simulink model "simlag2"  (Simulink 7.9)
settings: Solver=ode45  StartTime=0.0  StopTime=10.0  RelTol=1e-3
undefined symbols (not defined in the file or in its folder): Ax, Ay, Az, b, g, Ixx, Iyy, Izz, k, l, m
settings Model: Creator=gabriel  LastModifiedBy=gabriel
settings DebuggingCC: SolverPrmCheckMsg=none

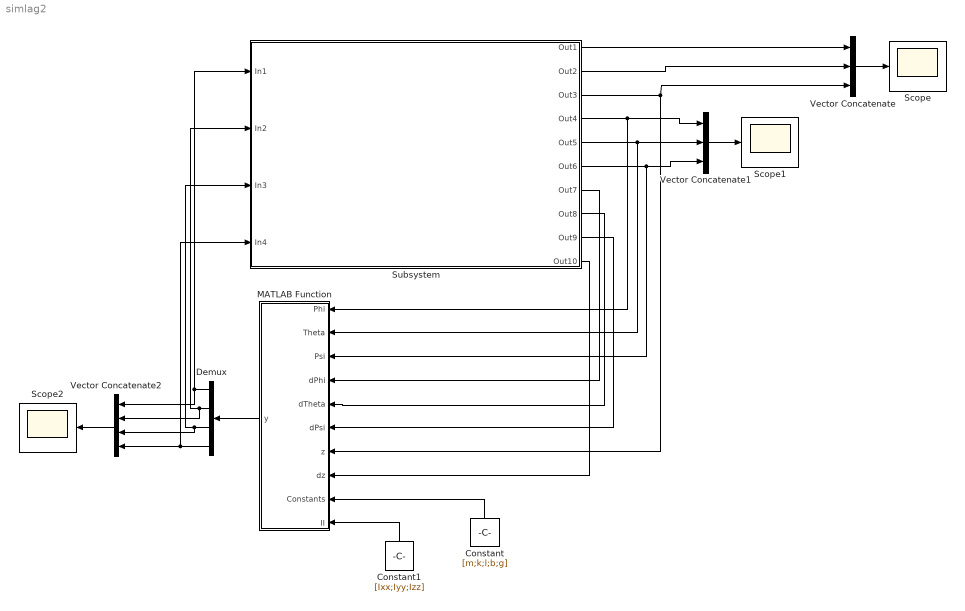
== system simlag2 ==
  Constant : Constant  Value=[m;k;l;b;g]
  Constant1 : Constant  Value=[Ixx;Iyy;Izz]
  Demux : Demux
  MATLAB Function : MATLAB Function  TreatAsAtomicUnit=on
  Scope : Scope
      settings: TickLabels=on  ShowLegends=on
  Scope1 : Scope
      settings: ShowLegends=on
  Scope2 : Scope
      settings: TickLabels=on  ShowLegends=on  SaveName=ScopeData2
  Subsystem : Subsystem
      mask Display: image(imread('Quad.jpeg'))
  Vector Concatenate : Concatenate  NumInputs=3
  Vector Concatenate1 : Concatenate  NumInputs=3
  Vector Concatenate2 : Concatenate  NumInputs=4
  wires:
  Subsystem/1(Out1) -> Vector Concatenate/1
  Subsystem/2(Out2) -> Vector Concatenate/2
  Subsystem/3(Out3) -> Vector Concatenate/3, MATLAB Function/7(z)
  Vector Concatenate/1 -> Scope/1
  Subsystem/4(Out4) -> Vector Concatenate1/1, MATLAB Function/1(Phi)
  Subsystem/5(Out5) -> Vector Concatenate1/2, MATLAB Function/2(Theta)
  Subsystem/6(Out6) -> Vector Concatenate1/3, MATLAB Function/3(Psi)
  Vector Concatenate1/1 -> Scope1/1
  Subsystem/7(Out7) -> MATLAB Function/4(dPhi)
  Subsystem/8(Out8) -> MATLAB Function/5(dTheta)
  Subsystem/9(Out9) -> MATLAB Function/6(dPsi)
  Subsystem/10(Out10) -> MATLAB Function/8(dz)
  Constant/1 -> MATLAB Function/9(Constants)
  Constant1/1 -> MATLAB Function/10(II)
  MATLAB Function/1(y) -> Demux/1
  Demux/1 -> Subsystem/1(In1), Vector Concatenate2/1
  Demux/2 -> Subsystem/2(In2), Vector Concatenate2/2
  Demux/3 -> Subsystem/3(In3), Vector Concatenate2/3
  Demux/4 -> Subsystem/4(In4), Vector Concatenate2/4
  Vector Concatenate2/1 -> Scope2/1

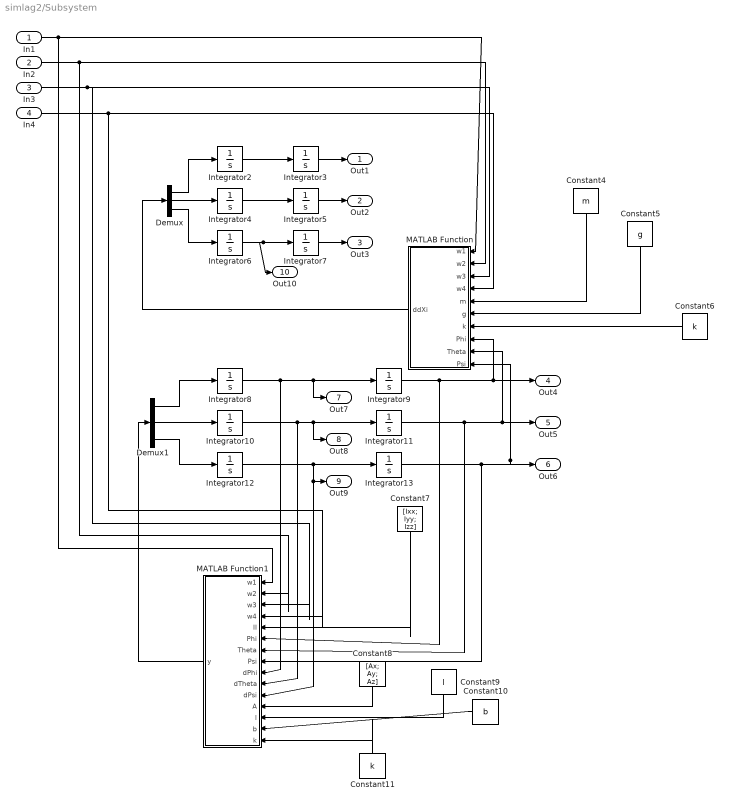
== system simlag2/Subsystem ==
  In1 : Inport
  In2 : Inport  Port=2
  In3 : Inport  Port=3
  In4 : Inport  Port=4
  Constant10 : Constant  Value=b
  Constant11 : Constant  Value=k
  Constant4 : Constant  Value=m
  Constant5 : Constant  Value=g
  Constant6 : Constant  Value=k
  Constant7 : Constant  Value=[Ixx; Iyy; Izz]
  Constant8 : Constant  Value=[Ax; Ay; Az]
  Constant9 : Constant  Value=l
  Demux : Demux  Outputs=3
  Demux1 : Demux  Outputs=3
  Integrator{2..13} (12 alike) : Integrator
  MATLAB Function : MATLAB Function  TreatAsAtomicUnit=on
  MATLAB Function1 : MATLAB Function  TreatAsAtomicUnit=on
  Out1 : Outport
  Out2 : Outport  Port=2
  Out3 : Outport  Port=3
  Out4 : Outport  Port=4
  Out5 : Outport  Port=5
  Out6 : Outport  Port=6
  Out7 : Outport  Port=7
  Out8 : Outport  Port=8
  Out9 : Outport  Port=9
  Out10 : Outport  Port=10
  wires:
  Integrator2/1 -> Integrator3/1
  Integrator4/1 -> Integrator5/1
  Integrator6/1 -> Integrator7/1, Out10/1
  Integrator8/1 -> MATLAB Function1/9(dPhi), Integrator9/1, Out7/1
  Integrator10/1 -> MATLAB Function1/10(dTheta), Integrator11/1, Out8/1
  Integrator12/1 -> Integrator13/1, MATLAB Function1/11(dPsi), Out9/1
  In1/1 -> MATLAB Function/1(w1), MATLAB Function1/1(w1)
  Integrator9/1 -> MATLAB Function1/6(Phi), MATLAB Function/8(Phi), Out4/1
  Integrator11/1 -> MATLAB Function1/7(Theta), MATLAB Function/9(Theta), Out5/1
  Integrator13/1 -> MATLAB Function1/8(Psi), MATLAB Function/10(Psi), Out6/1
  Constant4/1 -> MATLAB Function/5(m)
  Constant5/1 -> MATLAB Function/6(g)
  Constant6/1 -> MATLAB Function/7(k)
  MATLAB Function/1(ddXi) -> Demux/1
  Demux/1 -> Integrator2/1
  Demux/2 -> Integrator4/1
  Demux/3 -> Integrator6/1
  Constant7/1 -> MATLAB Function1/5(II)
  Demux1/1 -> Integrator8/1
  Demux1/2 -> Integrator10/1
  Demux1/3 -> Integrator12/1
  MATLAB Function1/1(y) -> Demux1/1
  Constant8/1 -> MATLAB Function1/12(A)
  Constant9/1 -> MATLAB Function1/13(l)
  Constant10/1 -> MATLAB Function1/14(b)
  Constant11/1 -> MATLAB Function1/15(k)
  Integrator3/1 -> Out1/1
  Integrator5/1 -> Out2/1
  Integrator7/1 -> Out3/1
  In2/1 -> MATLAB Function/2(w2), MATLAB Function1/2(w2)
  In3/1 -> MATLAB Function/3(w3), MATLAB Function1/3(w3)
  In4/1 -> MATLAB Function/4(w4), MATLAB Function1/4(w4)

== matlab function Subsystem/MATLAB Function1 ==
  data: w1 input double; w2 input double; w3 input double; w4 input double; y output double; II input double; Phi input double; Theta input double; Psi input double; dPhi input double; dTheta input double; dPsi input double; A input double; l input double; b input double; k input double
function y = fcn(w1,w2,w3,w4,II,Phi,Theta,Psi,dPhi,dTheta,dPsi,A,l,b,k)
%#codegen

Ixx=II(1);
Iyy=II(2);
Izz=II(3);

% TauB=[[l*k*(w(4)^2-w(2)^2)];
%       [l*k*(w(3)^2-w(1)^2)];
%       [b*(w(1)^2+w(3)^2-w(2)^2-w(4)^2)]];

TauB=[[l*k*(w4-w2)];
      [l*k*(w3-w1)];
      [b*(w1+w3-w2-w4)]];

Weta=[[1 0 -sin(Theta)];
      [0 cos(Phi) cos(Theta)*sin(Phi)];
      [0 -sin(Phi) cos(Theta)*cos(Phi)]];
 
J=transpose(Weta)*[[Ixx 0 0];[0 Iyy 0];[0 0 Izz]]*Weta;  

% CdEta=[((Izz*sin(2*Phi)*cos(Theta)^2)/2 - (Iyy*sin(2*Phi)*cos(Theta)^2)/2)*dPsi^2 + (Izz*cos(2*Phi)*cos(Theta) - Iyy*cos(2*Phi)*cos(Theta) - Ixx*cos(Theta))*dPsi*dTheta + ((Iyy*sin(2*Phi))/2 - (Izz*sin(2*Phi))/2)*dTheta^2;
%        dPsi^2*(Izz*cos(Phi)^2*cos(Theta)*sin(Theta) - Ixx*cos(Theta)*sin(Theta) + Iyy*cos(Theta)*sin(Phi)^2*sin(Theta)) - ddTheta*(Iyy*cos(Phi)^2 + Izz*sin(Phi)^2) - ddPsi*(Iyy*cos(Phi)*cos(Theta)*sin(Phi) - Izz*cos(Phi)*cos(Theta)*sin(Phi)) + Iyy*ddTheta*cos(Phi)^2 + Izz*ddTheta*sin(Phi)^2 - dPhi*dTheta*(2*Iyy*cos(Phi)*sin(Phi) - 2*Izz*cos(Phi)*sin(Phi)) + dPhi*dPsi*(Ixx*cos(Theta) + Iyy*cos(Phi)^2*cos(Theta) - Izz*cos(Phi)^2*cos(Theta) - Iyy*cos(Theta)*sin(Phi)^2 + Izz*cos(Theta)*sin(Phi)^2) + Iyy*ddPsi*cos(Phi)*cos(Theta)*sin(Phi) - Izz*ddPsi*cos(Phi)*cos(Theta)*sin(Phi);
%        Ixx*ddPsi*sin(Theta)^2 - ddPsi*(Izz*cos(Phi)^2*cos(Theta)^2 + Iyy*cos(Theta)^2*sin(Phi)^2 + Ixx*sin(Theta)^2) - ddTheta*(Iyy*cos(Phi)*cos(Theta)*sin(Phi) - Izz*cos(Phi)*cos(Theta)*sin(Phi)) - dTheta^2*(Iyy*cos(Phi)*sin(Phi)*sin(Theta) - Izz*cos(Phi)*sin(Phi)*sin(Theta)) - dPsi*dTheta*(2*Izz*cos(Phi)^2*cos(Theta)*sin(Theta) - 2*Ixx*cos(Theta)*sin(Theta) + 2*Iyy*cos(Theta)*sin(Phi)^2*sin(Theta)) - dPhi*dTheta*(Ixx*cos(Theta) - Iyy*cos(Phi)^2*cos(Theta) + Izz*cos(Phi)^2*cos(Theta) + Iyy*cos(Theta)*sin(Phi)^2 - Izz*cos(Theta)*sin(Phi)^2) + dPhi*dPsi*(2*Iyy*cos(Phi)*cos(Theta)^2*sin(Phi) - 2*Izz*cos(Phi)*cos(Theta)^2*sin(Phi)) + Izz*ddPsi*cos(Phi)^2*cos(Theta)^2 + Iyy*ddPsi*cos(Theta)^2*sin(Phi)^2 + Iyy*ddTheta*cos(Phi)*cos(Theta)*sin(Phi) - Izz*ddTheta*cos(Phi)*cos(Theta)*sin(Phi)]
 
% CdEta=[(Iyy*dTheta^2*sin(2*Phi))/2 - (Izz*dTheta^2*sin(2*Phi))/2 - Ixx*dPsi*dTheta*cos(Theta) - (Iyy*dPsi^2*sin(2*Phi)*cos(Theta)^2)/2 + (Izz*dPsi^2*sin(2*Phi)*cos(Theta)^2)/2 - Iyy*dPsi*dTheta*cos(2*Phi)*cos(Theta) + Izz*dPsi*dTheta*cos(2*Phi)*cos(Theta);
%         dPhi*(Ixx*dPsi*cos(Theta) - 2*Iyy*dTheta*cos(Phi)*sin(Phi) + 2*Izz*dTheta*cos(Phi)*sin(Phi) + Iyy*dPsi*cos(Phi)^2*cos(Theta) - Izz*dPsi*cos(Phi)^2*cos(Theta) - Iyy*dPsi*cos(Theta)*sin(Phi)^2 + Izz*dPsi*cos(Theta)*sin(Phi)^2) - Ixx*dPsi^2*cos(Theta)*sin(Theta) + Iyy*dPsi^2*cos(Theta)*sin(Phi)^2*sin(Theta) + Izz*dPsi^2*cos(Phi)^2*cos(Theta)*sin(Theta);
%         -dPhi*(Ixx*dTheta*cos(Theta) - Iyy*dTheta*cos(Phi)^2*cos(Theta) + Izz*dTheta*cos(Phi)^2*cos(Theta) + Iyy*dTheta*cos(Theta)*sin(Phi)^2 - Izz*dTheta*cos(Theta)*sin(Phi)^2 - 2*Iyy*dPsi*cos(Phi)*cos(Theta)^2*sin(Phi) + 2*Izz*dPsi*cos(Phi)*cos(Theta)^2*sin(Phi))  - Iyy*dTheta^2*cos(Phi)*sin(Phi)*sin(Theta) + Izz*dTheta^2*cos(Phi)*sin(Phi)*sin(Theta) + 2*Ixx*dPsi*dTheta*cos(Theta)*sin(Theta) - 2*Izz*dPsi*dTheta*cos(Phi)^2*cos(Theta)*sin(Theta) - 2*Iyy*dPsi*dTheta*cos(Theta)*sin(Phi)^2*sin(Theta)];    


  CdEta=[(Iyy*dTheta^2*sin(2*Phi))/2 - (Izz*dTheta^2*sin(2*Phi))/2 - Ixx*dPsi*dTheta*cos(Theta) - (Iyy*dPsi^2*sin(2*Phi)*cos(Theta)^2)/2 + (Izz*dPsi^2*sin(2*Phi)*cos(Theta)^2)/2 - Iyy*dPsi*dTheta*cos(2*Phi)*cos(Theta) + Izz*dPsi*dTheta*cos(2*Phi)*cos(Theta);
          dPhi*(Ixx*dPsi*cos(Theta) - 2*Iyy*dTheta*cos(Phi)*sin(Phi) + 2*Izz*dTheta*cos(Phi)*sin(Phi) + Iyy*dPsi*cos(Phi)^2*cos(Theta) - Izz*dPsi*cos(Phi)^2*cos(Theta) - Iyy*dPsi*cos(Theta)*sin(Phi)^2 + Izz*dPsi*cos(Theta)*sin(Phi)^2)  - Ixx*dPsi^2*cos(Theta)*sin(Theta) + Iyy*dPsi^2*cos(Theta)*sin(Phi)^2*sin(Theta)  + Izz*dPsi^2*cos(Phi)^2*cos(Theta)*sin(Theta);
          -dPhi*(Ixx*dTheta*cos(Theta) - Iyy*dTheta*cos(Phi)^2*cos(Theta) + Izz*dTheta*cos(Phi)^2*cos(Theta) + Iyy*dTheta*cos(Theta)*sin(Phi)^2 - Izz*dTheta*cos(Theta)*sin(Phi)^2 - 2*Iyy*dPsi*cos(Phi)*cos(Theta)^2*sin(Phi) + 2*Izz*dPsi*cos(Phi)*cos(Theta)^2*sin(Phi))  - Iyy*dTheta^2*cos(Phi)*sin(Phi)*sin(Theta) + Izz*dTheta^2*cos(Phi)*sin(Phi)*sin(Theta) + 2*Ixx*dPsi*dTheta*cos(Theta)*sin(Theta) - 2*Izz*dPsi*dTheta*cos(Phi)^2*cos(Theta)*sin(Theta) - 2*Iyy*dPsi*dTheta*cos(Theta)*sin(Phi)^2*sin(Theta)];
y = inv(J)*(TauB-CdEta);

== matlab function Subsystem/MATLAB Function ==
  data: w1 input double; w2 input double; w3 input double; w4 input double; m input double; g input double; k input double; Phi input double; Theta input double; Psi input double; ddXi output double
function ddXi = fcn(w1,w2,w3,w4,m,g,k,Phi,Theta,Psi)
%#codegen

R=[[cos(Psi)*cos(Theta) cos(Psi)*sin(Theta)*sin(Phi)-sin(Psi)*cos(Phi) cos(Psi)*sin(Theta)*cos(Phi)+sin(Psi)*sin(Phi)];
   [sin(Psi)*cos(Theta) sin(Psi)*sin(Theta)*sin(Phi)+cos(Psi)*cos(Phi) sin(Psi)*sin(Theta)*cos(Phi)-cos(Psi)*sin(Phi)];
   [-sin(Theta) cos(Theta)*sin(Phi) cos(Theta)*cos(Phi)]];

% T=[0; 0; k*(w(1)^2+w(2)^2+w(3)^2+w(4)^2)/m];

T=[0; 0; k*(w1+w2+w3+w4)/m];

ddXi = R*T+[0; 0; -g];

== matlab function MATLAB Function ==
  data: Phi input double; y output double; Theta input double; Psi input double; dPhi input double; dTheta input double; dPsi input double; z input double; dz input double; Constants input double; II input double
function y = fcn(Phi,Theta,Psi,dPhi,dTheta,dPsi,z,dz,Constants,II)
%#codegen

m=Constants(1);
k=Constants(2);
l=Constants(3);
b=Constants(4);
g=Constants(5);

Ixx=II(1);
Iyy=II(2);
Izz=II(3);

zD=10;
dzD=0;

PhiD=0.5;
ThetaD=0;
PsiD=0;

dPhiD=0;
dThetaD=0;
dPsiD=0;

KphiP=1.5;
KthetaP=6;
KpsiP=6;
KzP=6;

KphiD=2.5;
KthetaD=1.75;
KpsiD=1.75;
KzD=1.75;

T=(g+KzD*(dzD-dz)+KzP*(zD-z))*m/(cos(Phi)*cos(Theta));

TauPhi=Ixx*(KphiD*(dPhiD-dPhi)+KphiP*(PhiD-Phi));

TauTheta=Iyy*(KthetaD*(dThetaD-dTheta)+KthetaP*(ThetaD-Theta));

TauPsi=Izz*(KpsiD*(dPsiD-dPsi)+KpsiP*(PsiD-Psi));

y = [(T/(4*k)-TauTheta/(2*k*l)-TauPsi/(4*b));
     (T/(4*k)-TauPhi/(2*k*l)+TauPsi/(4*b));
     (T/(4*k)+TauTheta/(2*k*l)-TauPsi/(4*b));
     (T/(4*k)+TauPhi/(2*k*l)+TauPsi/(4*b))];
